simulink model "Project_One_Simulink"  (R2018b)
settings: Solver=VariableStepAuto  StartTime=0.0  StopTime=25  MaxStep=1e-4  RelTol=1e-3
values from neighbouring files (symbols this model uses):
  b = 220    [Project_One.m]
  b1 = 170    [Project_One.m]
  b2 = 10    [Project_One.m]
  f = 2*pi*v/L    (= 194.45781875)    [Project_One.m]    (also in gui_try.m = 2*pi*v/0.65)
  k = 25000    [Project_One.m]
  k1 = 4000    [Project_One.m]
  k2 = 6000    [Project_One.m]
  m = 150    [Project_One.m]
  m1 = 125    [Project_One.m]
  m2 = 75    [Project_One.m]
  p = 2*f    (= 388.9156375)    [Project_One.m]    (also in gui_try.m = 2*f)
  TT = 2+3*(2*pi/f)    (= 2.09693390599)    [Project_One.m]    (also in gui_try.m = 2+3*(2*pi/f))
settings Model: Creator=cipher  LastModifiedBy=cipher

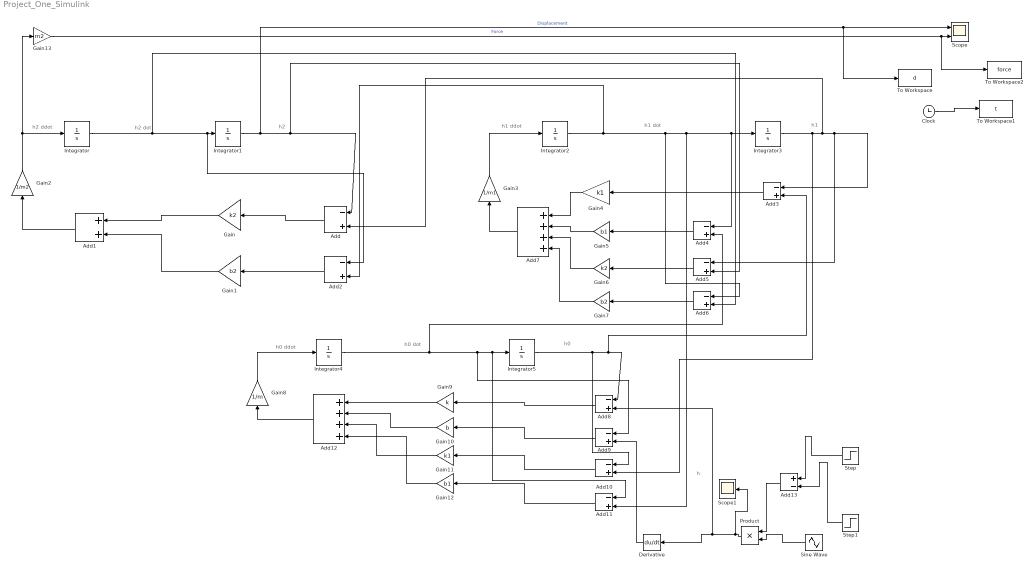
== system Project_One_Simulink ==
  note: h
  note: h0
  note: h0 ddot
  note: h1
  note: h1 ddot
  note: h1 dot
  note: h2 ddot
  note: h2
  note: h2 dot
  note: h0 dot
  Add{,2..6,8..11} (10 alike) : Sum  Inputs=-+
  Add1 : Sum
  Add12 : Sum  Inputs=++++
  Add13 : Sum  Inputs=+-
  Add7 : Sum  Inputs=++++
  Clock : Clock
  Derivative : Derivative
  Gain : Gain  Gain=k2
  Gain1 : Gain  Gain=b2
  Gain10 : Gain  Gain=b
  Gain11 : Gain  Gain=k1
  Gain12 : Gain  Gain=b1
  Gain13 : Gain  Gain=m2
  Gain2 : Gain  Gain=1/m2
  Gain3 : Gain  Gain=1/m1
  Gain4 : Gain  Gain=k1
  Gain5 : Gain  Gain=b1
  Gain6 : Gain  Gain=k2
  Gain7 : Gain  Gain=b2
  Gain8 : Gain  Gain=1/m
  Gain9 : Gain  Gain=k
  Integrator{,1..5} (6 alike) : Integrator
  Product : Product
  Scope : Scope  NumInputPorts=2
  Scope1 : Scope
  Sine Wave : Sin  Amplitude=0.35  Frequency=f  Phase=-p  SampleTime=0
  Step : Step  Time=2  SampleTime=0
  Step1 : Step  Time=TT  SampleTime=0
  To Workspace : ToWorkspace  VariableName=d  SampleTime=-1
  To Workspace1 : ToWorkspace  VariableName=t  SampleTime=-1
  To Workspace2 : ToWorkspace  VariableName=force  SampleTime=-1
  wires:
  Integrator/1 -> Add6/2, Add2/1, Integrator1/1
  Integrator1/1 -> To Workspace/1, Scope/1, Add5/2, Add/1  "Displacement"
  Add/1 -> Gain/1
  Gain1/1 -> Add1/2
  Gain/1 -> Add1/1
  Add1/1 -> Gain2/1
  Gain2/1 -> Gain13/1, Integrator/1
  Add2/1 -> Gain1/1
  Integrator2/1 -> Add2/2, Add6/1, Add4/1, Integrator3/1, Add11/2
  Gain3/1 -> Integrator2/1
  Integrator3/1 -> Add10/2, Add/2, Add5/1, Add3/1
  Add3/1 -> Gain4/1
  Add4/1 -> Gain5/1
  Add5/1 -> Gain6/1
  Add6/1 -> Gain7/1
  Gain4/1 -> Add7/1
  Gain5/1 -> Add7/2
  Gain6/1 -> Add7/3
  Gain7/1 -> Add7/4
  Add7/1 -> Gain3/1
  Gain8/1 -> Integrator4/1
  Integrator5/1 -> Add10/1, Add3/2, Add8/1
  Add8/1 -> Gain9/1
  Add9/1 -> Gain10/1
  Add10/1 -> Gain11/1
  Add11/1 -> Gain12/1
  Gain9/1 -> Add12/1
  Gain10/1 -> Add12/2
  Gain11/1 -> Add12/3
  Gain12/1 -> Add12/4
  Add12/1 -> Gain8/1
  Integrator4/1 -> Add4/2, Add11/1, Integrator5/1, Add9/1
  Derivative/1 -> Add9/2
  Sine Wave/1 -> Product/2
  Product/1 -> Scope1/1, Add8/2, Derivative/1
  Step/1 -> Add13/1
  Step1/1 -> Add13/2
  Add13/1 -> Product/1
  Gain13/1 -> To Workspace2/1, Scope/2  "Force"
  Clock/1 -> To Workspace1/1
